simulink model "Link_B_org"  (Simulink 10.0)
settings: Solver=FixedStepAuto  StartTime=0.0  StopTime=15  FixedStep=1  RelTol=1e-3
model workspace (MAT data in the model file):
  Var : num (value not decoded)
libraries: Blocks_Lib x9
settings Model: Creator=aw5670  LastModifiedBy=bhisma
settings DataIOCC: LimitDataPoints=on
settings OptimizationCC: BlockReduction=off  BooleanDataType=off
settings DebuggingCC: SaveWithParameterizedLinksMsg=none  SignalResolutionControl=TryResolveAllWithWarning
settings HardwareCC: TargetUnknown=on
settings GRTTargetCC: GeneratePreprocessorConditionals=Disable all  CombineOutputUpdateFcns=on  GRTInterface=off
settings ConfigComp: CovExternalEMLEnable=off  CovSFcnEnable=off

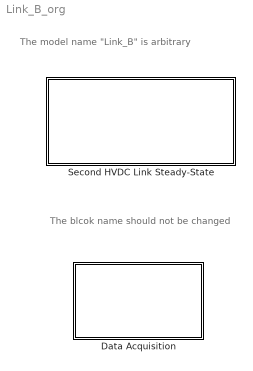
== system Link_B_org ==
  note: The model name "Link_B" is arbitrary
  note: The blcok name should not be changed
  Data Acquisition : Subsystem  mask{Ts=1}
      mask prompts: Ts "Sample time :"
      mask Display: disp('Open this block\nto visualize\nrecorded signals')
  Second HVDC Link Steady-State : Subsystem  mask(HVDC link steady-state model){NB_R=2, NOT_USED_3=, NOT_USED_4=, Pn_R=600, U1_R=[735, 0.0025, 0.01], U2_R=[200, 0.0025, 0.11], NOT_USED_0=DC current, NOT_USED_1=0, AMODE_ANGLE=5, LOCK_TAP_R=off, TCC_UDI0_MODE_R=off, ANGLE_R=[14.0, 17.0], Udi0_ref_R=280, TSTP_R=0.0125, TAP_R=[0.9375, 1.125], TAP_R_INI=1, Eac_R_INI=735, NB_I=2, NOT_USED_5=, NOT_USED_6=, Pn_I=600, U1_I=[735, 0.0025, 0.01], U2_I=[200, 0.0025, 0.11], C_MODE_I=DC voltage, GAMMA_REF=22, VSCHED=500, GMODE_ANGLE=17, NOT_USED_2=0, LOCK_TAP_I=off, TCC_UDI0_MODE_I=off, ANGLE_I=[20.0, 23.0], Udi0_ref_I=280, TSTP_I=0.0125, TAP_I=[0.9125, 1.0875], TAP_I_INI=1, Eac_I_INI=735, RDC=12.0 + 2*0.3, RCOMP=0.3, MC_MODE=Power, SLACK_ST=Rectifier, SETVAL_MW=100, SETVAL_kA=1, VCMODE=500*0.94, DELTI=0.2, Tap_pu_R_B=0.9875, Eac_R_B=741.9693, Udi0_R_B=276.1073, Tap_limited_R_B=0, alpha_R_B=16.7041, Idc_R_B=1, Vdc_R_B=512.3, Pdc_R_B=512.3, Pac_R_B=513.6333, Qac_R_B=201.3195, Tap_pu_I_B=1.0125, Eac_I_B=760.915, Udi0_I_B=276.166, Tap_limited_I_B=0, alpha_I_B=151.0016, gamma_I_B=21.5717, Vdc_I_B=499.7, Pdc_I_B=-499.7, Pac_I_B=-498.3667, Qac_I_B=237.2282, DC_iter_B=2, Ts=1}
      mask prompts: NB_R "Number of 6 pulse converter units in series"; NOT_USED_3 "AC bus name"; NOT_USED_4 "PQ load name"; Pn_R "Power (MVA)"; U1_R "Primary winding (AC side) parameters [V1 Ph-Ph(kVrms), R1(pu), L1(pu)]"; U2_R "Secondary winding (DC side) parameters [V2 Ph-Ph(kVrms), R2(pu), L2(pu)]"; NOT_USED_0 "Control mode"; NOT_USED_1 "not used"; AMODE_ANGLE "Minimum alpha (deg.)"; LOCK_TAP_R "Lock tap ratio"; TCC_UDI0_MODE_R "Udi0 control mode"; ANGLE_R "Angle range [min, max] (deg.)"; Udi0_ref_R "Udi0 reference (kV)"; TSTP_R "Tap step size (pu)"; TAP_R "Tap range [min, max] (pu)"; TAP_R_INI "Tap ratio (pu)"; Eac_R_INI "Primary AC voltage  (Ph-Ph(kVrms))"; NB_I "Number of 6 pulse converter units in series"; NOT_USED_5 "AC bus name"; NOT_USED_6 "PQ load name"; Pn_I "Power (MVA)"; U1_I "Primary winding (AC side) parameters [V1 Ph-Ph(kVrms), R1(pu), L1(pu)]"; U2_I "Secondary winding (DC side) parameters [V2 Ph-Ph(kVrms), R2(pu), L2(pu)]"; C_MODE_I "Control mode"; GAMMA_REF "Gamma reference (deg.)"; VSCHED "Voltage reference (kV)"; GMODE_ANGLE "Minimum gamma (deg.)"; NOT_USED_2 "Not used"; LOCK_TAP_I "Lock tap ratio"; TCC_UDI0_MODE_I "Udi0 control mode"; ANGLE_I "Angle range  [min, max] (deg.)"; Udi0_ref_I "Udi0 reference (kV)"; TSTP_I "Tap step size (pu)"; TAP_I "Tap range [min, max] (pu)"; TAP_I_INI "Tap ratio (pu)"; Eac_I_INI "Primary AC voltage  (Ph-Ph(kVrms))"; RDC "Total link resistance (ohm)"; RCOMP "Resistance between voltage measurement and converter (ohm)"; MC_MODE "Control mode"; SLACK_ST "Slack station"; SETVAL_MW "Power reference (MW)"; SETVAL_kA "Current reference (kA)"; VCMODE "Inverter DC voltage threshold in power control (kV)"; DELTI "Inverter current margin (kA)"; Tap_pu_R_B "Tap ratio (pu)"; Eac_R_B "Eac (kV)"; Udi0_R_B "Udi0 (kV)"; Tap_limited_R_B "Tap is limited"; alpha_R_B "Alpha (deg.)"; Idc_R_B "Idc (kA)"; Vdc_R_B "Vdc (kV)"; Pdc_R_B "Pdc (MW)"; Pac_R_B "Pac (MW)"; Qac_R_B "Qac (Mvar)"; Tap_pu_I_B "Tap ratio (pu)"; Eac_I_B "Eac (kV)"; Udi0_I_B "Udi0 (kV)"; Tap_limited_I_B "Tap is limited"; alpha_I_B "Alpha (deg.)"; gamma_I_B "Gamma (deg.)"; Vdc_I_B "Vdc (kV)"; Pdc_I_B "Pdc (MW)"; Pac_I_B "Pac (MW)"; Qac_I_B "Qac (Mvar)"; DC_iter_B "Iterations"; Ts "Sample time :"
      mask help: Implements a steady state model of a two terminal HVDC link for the DC load flow solution.
      mask init:
      | % History values 
      | Eac_R_B     = Eac_R_INI;
      | Eac_I_B     = Eac_I_INI;
      | TAPINI_R_B  = TAP_R_INI;
      | TAPINI_I_B  = TAP_I_INI;
      | 
      | % --- RECTIFIER ---
      | 
      | % Primary
      | V1_R = U1_R(1);
      | R1_R = U1_R(2);
      | L1_R = U1_R(3);
      | 
      | % Secondary
      | V2_R = U2_R(1);
      | R2_R = U2_R(2);
      | L2_R = U2_R(3);
      | 
      | % Nominal turn ratio (Usec/Uprim):
      | TR_R = V2_R/V1_R;
      | 
      | % Transformer reactance seen from secondary, per bridge [XC](ohm):
      | XC_R = (L1_R+L2_R)*V2_R^2/Pn_R;
      | 
      | % Transformer resistance seen from secondary, per bridge [RC](ohm):
      | RC_R = (R1_R+R2_R)* V2_R^2/Pn_R; 
      | 
      | % Tap Changer Control
      | ALFMIN_R=ANGLE_R(1);
      | ALFMAX_R=ANGLE_R(2);
      | 
      | TAPMN_R=TAP_R(1);
      | TAPMX_R=TAP_R(2);
      | 
      | % --- INVERTER ---
      | % Primary
      | V1_I = U1_I(1);
      | R1_I = U1_I(2);
      | L1_I = U1_I(3);
      | 
      | % Secondary
      | V2_I = U2_I(1);
      | R2_I = U2_I(2);
      | L2_I = U2_I(3);
      | 
      | % Nominal turn ratio (Usec/Uprim):
      | TR_I = V2_I/V1_I;
      | 
      | % Transformer reactance seen from secondary, per bridge [XC](ohm):
      | XC_I = (L1_I+L2_I)*V2_I^2/Pn_I;
      | 
      | % Transformer resistance seen from secondary, per bridge [RC](ohm):
      | RC_I = (R1_I+R2_I)* V2_I^2/Pn_I; 
      | 
      | % Pole Control
      | GC = C_MODE_I - 1;  % GC (0/1) is used in the model
      | 
      | % Tap Changer Control
      | GAMMIN_I=ANGLE_I(1);
      | GAMMAX_I=ANGLE_I(2);
      | 
      | TAPMN_I=TAP_I(1);
      | TAPMX_I=TAP_I(2);
      | 
      | DCVMIN_I   = VSCHED * (1 - TSTP_I);     %(kV)
      | DCVMAX_I   = VSCHED * (1 + TSTP_I);
      | 
      | % --- Master Control ---
      | MDC = MC_MODE - 1;     % MDC (0,1, or 2) used in the model 
      | 
      | if (MDC == 1)   
      |     SETVAL = SETVAL_MW;
      | elseif (MDC == 2)
      |     SETVAL = SETVAL_kA;
      | else
      |     SETVAL = 0;
      | end
      mask Help: web('HVDC_Link_SS_help.htm');
      mask TypeOptions NOT_USED_0: DC current
      mask Callback LOCK_TAP_R:
      | mode=get_param(gcb,'LOCK_TAP_R');
      | cb = get_param(gcb,'MaskEnables');
      | cb{11}='on'; cb{12}='on';
      | 
      | if strcmp(mode,'on')
      |  cb{11}='off';  % Udi0 control mode
      |  cb{12}='off';  % Angle range
      | end
      | 
      | set_param(gcb,'MaskEnables',cb);
      mask Callback TCC_UDI0_MODE_R:
      | mode=get_param(gcb,'TCC_UDI0_MODE_R');
      | cb = get_param(gcb,'MaskEnables');
      | cb{10}='on'; cb{12}='on'; cb{13}='off';
      | 
      | if strcmp(mode,'on')
      |  cb{12}='off';  % Angle range
      |  cb{10}='off';  % Lock the tap position
      |  cb{13}='on';  % Lock the tap position
      | end
      | 
      | set_param(gcb,'MaskEnables',cb);
      mask TypeOptions C_MODE_I: DC voltage | Gamma angle
      mask Callback C_MODE_I:
      | mode=get_param(gcb,'C_MODE_I');
      | cb = get_param(gcb,'MaskEnables');
      | cb{25}='on'; cb{26}='on'; cb{27}='on'; cb{31}='on';
      | 
      | if strcmp(mode,'Gamma angle')
      |  cb{26}='off';    % Voltage reference
      |  cb{27}='off';    % Minimum gamma
      |  cb{31}='off';    % Angle range (gamma_
      | else
      |  cb{25}='off';    % Gamma reference
      | end
      | 
      | set_param(gcb,'MaskEnables',cb);
      mask Callback LOCK_TAP_I:
      | mode=get_param(gcb,'LOCK_TAP_I');
      | cb = get_param(gcb,'MaskEnables');
      | cb{30}='on'; cb{31}='on';
      | 
      | if strcmp(mode,'on')
      |  cb{30}='off';  % Udi0 control mode
      |  cb{31}='off';  % Angle range
      | end
      | 
      | set_param(gcb,'MaskEnables',cb);
      mask Callback TCC_UDI0_MODE_I:
      | mode=get_param(gcb,'TCC_UDI0_MODE_I');
      | cb = get_param(gcb,'MaskEnables');
      | cb{29}='on'; cb{31}='on';  cb{32}='off';
      | 
      | if strcmp(mode,'on')
      |  cb{29}='off';  % Lock the tap position
      |  cb{31}='off';  % Angle range
      |  cb{32}='on';   % Udi0 reference
      | end
      | 
      | set_param(gcb,'MaskEnables',cb);
      mask TypeOptions MC_MODE: Blocked | Power | Current
      mask Callback MC_MODE:
      | mode=get_param(gcb,'MC_MODE');
      | cb = get_param(gcb,'MaskEnables');
      |  cb{40}='on'; cb{41}='on'; cb{42}='on'; cb{43}='on';
      | 
      | if strcmp(mode,'Current')
      |  cb{40}='off';     % Slack station
      |  cb{41}='off';     % Power reference
      |  cb{43}='off';     % Inverter DC ...
      | end
      | 
      | if strcmp(mode,'Power')
      |  cb{42}='off';     % Current reference
      | end
      | 
      | set_param(gcb,'MaskEnables',cb);
      | clear cb mode;
      mask TypeOptions SLACK_ST: Rectifier | Inverter
      mask DialogControl Update_tap_R Prompt: Update
      mask DialogControl Update_tap_R Callback:
      | set_param(gcb,'TAP_R_INI',[num2str(Tap_pu_R(end)), '  %Updated']);
      | 
      | % Reset output values
      | set_param(gcb,'Idc_R',[num2str(0)]);
      | set_param(gcb,'alpha_R',[num2str(0)]);
      | set_param(gcb,'Udi0_R',[num2str(0)]);
      | set_param(gcb,'Vdc_R',[num2str(0)]);
      | set_param(gcb,'Pac_R',[num2str(0)]);
      | set_param(gcb,'Qac_R',[num2str(0)]);
      | set_param(gcb,'Pdc_R',[num2str(0)]);
      mask DialogControl Update_tap_I Prompt: Update
      mask DialogControl Update_tap_I Callback:
      | set_param(gcb,'TAP_I_INI',[num2str(Tap_pu_I(end)), '  %Updated']);
      | 
      | % Reset output values
      | set_param(gcb,'gamma_I',[num2str(0)]);
      | set_param(gcb,'alpha_I',[num2str(0)]);
      | set_param(gcb,'Udi0_I',[num2str(0)]);
      | set_param(gcb,'Vdc_I',[num2str(0)]);
      | set_param(gcb,'Pdc_I',[num2str(0)]);
      | set_param(gcb,'Pac_I',[num2str(0)]);
      | set_param(gcb,'Qac_I',[num2str(0)]);
      mask DialogControl Container31 Prompt: Rectifier
      mask DialogControl Container33 Prompt: Inverter
      mask DialogControl Control4 Prompt: Compute and Update
      mask DialogControl Control4 Callback:
      | sim(gcs);
      | set_param(gcb,'DC_iter_B',[num2str(DC_iter_B(end))]);
      | % Rectifier
      | set_param(gcb,'Eac_R_B',[num2str(Eac_R_B(end))]);
      | set_param(gcb,'Tap_pu_R_B',[num2str(Tap_pu_R_B(end))]);
      | set_param(gcb,'Tap_limited_R_B',[num2str(Tap_limited_R_B(end))]);
      | set_param(gcb,'Idc_R_B',[num2str(Idc_R_B(end))]);
      | set_param(gcb,'alpha_R_B',[num2str(alpha_R_B(end))]);
      | set_param(gcb,'Udi0_R_B',[num2str(Udi0_R_B(end))]);
      | set_param(gcb,'Vdc_R_B',[num2str(Vdc_R_B(end))]);
      | set_param(gcb,'Pdc_R_B',[num2str(Pdc_R_B(end))]);
      | set_param(gcb,'Pac_R_B',[num2str(Pac_R_B(end))]);
      | set_param(gcb,'Qac_R_B',[num2str(Qac_R_B(end))]);
      | 
      | % Inverter
      | set_param(gcb,'Eac_I_B',[num2str(Eac_I_B(end))]);
      | set_param(gcb,'Tap_pu_I_B',[num2str(Tap_pu_I_B(end))]);
      | set_param(gcb,'Tap_limited_I_B',[num2str(Tap_limited_I_B(end))]);
      | set_param(gcb,'gamma_I_B',[num2str(gamma_I_B(end))]);
      | set_param(gcb,'alpha_I_B',[num2str(alpha_I_B(end))]);
      | set_param(gcb,'Udi0_I_B',[num2str(Udi0_I_B(end))]);
      | set_param(gcb,'Vdc_I_B',[num2str(Vdc_I_B(end))]);
      | set_param(gcb,'Pdc_I_B',[num2str(Pdc_I_B(end))]);
      | set_param(gcb,'Pac_I_B',[num2str(Pac_I_B(end))]);
      | set_param(gcb,'Qac_I_B',[num2str(Qac_I_B(end))]);
      mask Display: disp('Steady-state model\nof HVDC link\n\n(for DC load flow solution)')

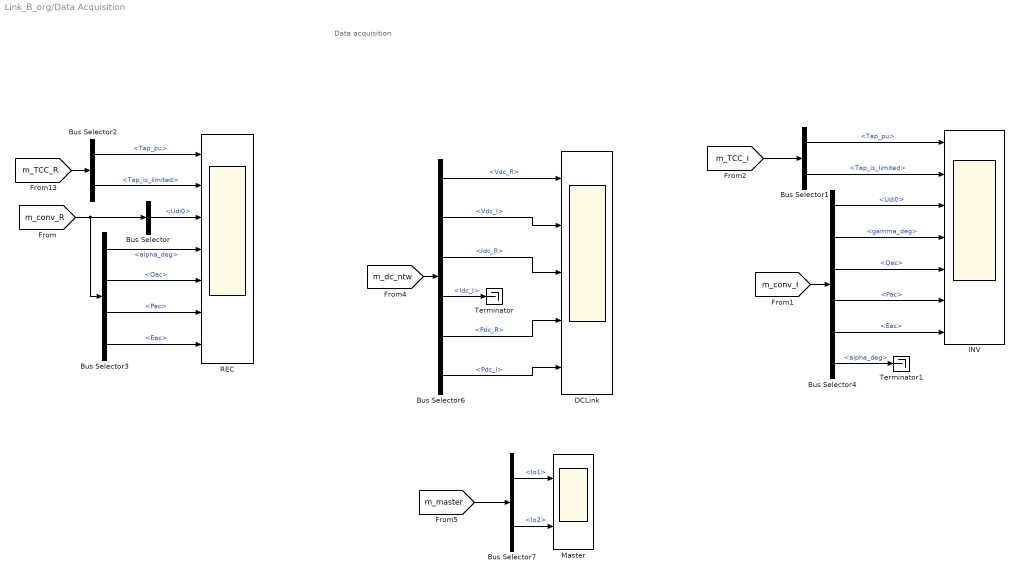
== system Link_B_org/Data Acquisition ==
  note: Data acquisition
  Bus Selector : BusSelector  OutputSignals=Udi0
  Bus Selector1 : BusSelector  OutputSignals=Tap_pu,Tap_is_limited
  Bus Selector2 : BusSelector  OutputSignals=Tap_pu,Tap_is_limited
  Bus Selector3 : BusSelector  OutputSignals=alpha_deg,Qac,Pac,Eac
  Bus Selector4 : BusSelector  OutputSignals=Udi0,gamma_deg,Qac,Pac,Eac,alpha_deg
  Bus Selector6 : BusSelector  OutputSignals=Vdc_R,Vdc_I,Idc_R,Idc_I,Pdc_R,Pdc_I
  Bus Selector7 : BusSelector  OutputSignals=Io1,Io2
  DCLink : Scope  NumInputPorts=5
  INV : Scope  NumInputPorts=7
  Master : Scope  NumInputPorts=2
  REC : Scope  NumInputPorts=7
  Terminator : Terminator
  Terminator1 : Terminator
  wires:
  Bus Selector1/1 -> INV/1  "<Tap_pu>"
  Bus Selector6/6 -> DCLink/5  "<Pdc_I>"
  Bus Selector6/5 -> DCLink/4  "<Pdc_R>"
  Bus Selector6/3 -> DCLink/3  "<Idc_R>"
  Bus Selector6/2 -> DCLink/2  "<Vdc_I>"
  Bus Selector1/2 -> INV/2  "<Tap_is_limited>"
  Bus Selector2/2 -> REC/2  "<Tap_is_limited>"
  Bus Selector7/2 -> Master/2  "<Io2>"
  Bus Selector7/1 -> Master/1  "<Io1>"
  [m_master] -> Bus Selector7/1
  Bus Selector/1 -> REC/3  "<Udi0>"
  [m_conv_R] -> Bus Selector/1, Bus Selector3/1
  Bus Selector3/2 -> REC/5  "<Qac>"
  Bus Selector3/1 -> REC/4  "<alpha_deg>"
  Bus Selector3/3 -> REC/6  "<Pac>"
  Bus Selector6/1 -> DCLink/1  "<Vdc_R>"
  Bus Selector2/1 -> REC/1  "<Tap_pu>"
  Bus Selector3/4 -> REC/7  "<Eac>"
  [m_conv_I] -> Bus Selector4/1
  [m_TCC_I] -> Bus Selector1/1
  [m_dc_ntw] -> Bus Selector6/1
  Bus Selector6/4 -> Terminator/1  "<Idc_I>"
  Bus Selector4/6 -> Terminator1/1  "<alpha_deg>"
  Bus Selector4/1 -> INV/3  "<Udi0>"
  Bus Selector4/2 -> INV/4  "<gamma_deg>"
  Bus Selector4/3 -> INV/5  "<Qac>"
  Bus Selector4/4 -> INV/6  "<Pac>"
  Bus Selector4/5 -> INV/7  "<Eac>"
  [m_TCC_R] -> Bus Selector2/1

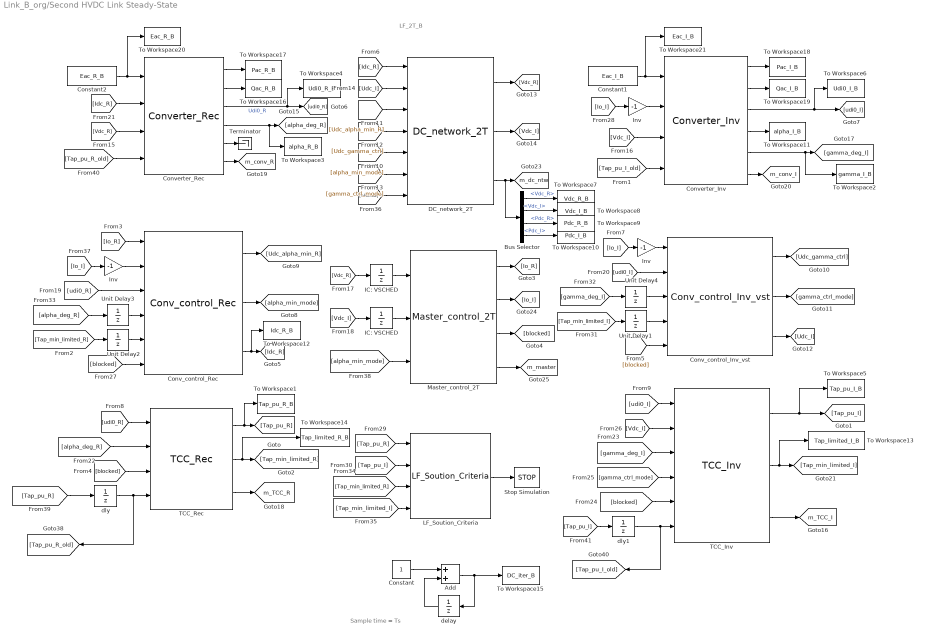
== system Link_B_org/Second HVDC Link Steady-State ==
  note: LF_2T_B
  note: Sample time = Ts
  " Inv " : Gain  Gain=-1
  Add : Sum
  Bus Selector : BusSelector  OutputSignals=Vdc_R,Vdc_I,Pdc_R,Pdc_I
  Constant : Constant
  Constant1 : Constant  Value=Eac_I_B
  Constant2 : Constant  Value=Eac_R_B
  Conv_control_Inv_vst : Blocks_Lib/Second HVDC Link Steady-State/Conv_control_Inv_vst  GC=GC  VSCHED=VSCHED  GMODE_ANGLE=GMODE_ANGLE  GAMMA_REF=GAMMA_REF  NB=NB_I  RC=RC_I  XC=XC_I
  Conv_control_Rec : Blocks_Lib/Second HVDC Link Steady-State/Conv_control_Rec  AMODE_ANGLE=AMODE_ANGLE  NB=NB_R  RC=RC_R  XC=XC_R
  Converter_Inv : Blocks_Lib/Second HVDC Link Steady-State/Converter_Inv  Pn=Pn_I  W1="[V1_I,  R1_I,  L1_I]"  W2=[V2_I, R2_I, L2_I]  TR=V2_I/V1_I  RC=(R1_I+R2_I)* V2_I^2/Pn_I;  XC=(L1_I+L2_I)*V2_I^2/Pn_I;  NB=NB_I
  Converter_Rec : Blocks_Lib/Second HVDC Link Steady-State/Converter_Rec  Pn=Pn_R  W1="[V1_R,  R1_R,  L1_R]"  W2="[V2_R,  R2_R,  L2_R]"  TR=V2_R/V1_R  RC=(R1_R+R2_R)* V2_R^2/Pn_R;  XC=(L1_R+L2_R)*V2_R^2/Pn_R;  NB=NB_R
  DC_network_2T : Blocks_Lib/Second HVDC Link Steady-State/DC_network_2T  RDC=RDC  RCOMP=RCOMP
  IC: VSCHED : UnitDelay  InitialCondition=VSCHED  SampleTime=-1  HasFrameUpgradeWarning=on
  "IC: VSCHED " : UnitDelay  InitialCondition=VSCHED  SampleTime=-1  HasFrameUpgradeWarning=on
  "Inv " : Gain  Gain=-1
  "Inv  " : Gain  Gain=-1
  LF_Soution_Criteria : Blocks_Lib/Second HVDC Link Steady-State/LF_Soution_Criteria
  Master_control_2T : Blocks_Lib/Second HVDC Link Steady-State/Master_control_2T  MDC=MDC  SLACK_ST=SLACK_ST  SETVAL=SETVAL  VCMODE=VCMODE
  Stop Simulation : Stop
  TCC_Inv : Blocks_Lib/Second HVDC Link Steady-State/TCC_Inv  LOCK_TAP=LOCK_TAP_I  TCC_UDI0_MODE=TCC_UDI0_MODE_I  Udi0_ref=Udi0_ref_I  TAPINI=TAPINI_I_B  TAPMN=TAPMN_I  TAPMX=TAPMX_I  TSTP=TSTP_I  GAMMIN=GAMMIN_I  GAMMAX=GAMMAX_I  DCVMIN=DCVMIN_I  DCVMAX=DCVMAX_I
      settings: AttributesFormatString=|
      | Udi0_min = (1-TSTP*0.75)* Udi0_ref
      | Udi0_max = (1+TSTP*0.75)* Udi0_ref
  TCC_Rec : Blocks_Lib/Second HVDC Link Steady-State/TCC_Rec  LOCK_TAP=LOCK_TAP_R  TCC_UDI0_MODE=TCC_UDI0_MODE_R  Udi0_ref=Udi0_ref_R  TAPINI=TAPINI_R_B  TAPMN=TAPMN_R  TAPMX=TAPMX_R  TSTP=TSTP_R  ALFMIN=ALFMIN_R  ALFMAX=ALFMAX_R
      settings: AttributesFormatString=|
      | Udi0_min = (1-TSTP*0.75)* Udi0_ref
      | Udi0_max = (1+TSTP*0.75)* Udi0_ref
  Terminator : Terminator
  To Workspace1 : ToWorkspace  VariableName=Tap_pu_R_B  SampleTime=-1
  To Workspace10 : ToWorkspace  VariableName=Pdc_I_B  SampleTime=-1
  To Workspace11 : ToWorkspace  VariableName=alpha_I_B  SampleTime=-1
  To Workspace12 : ToWorkspace  VariableName=Idc_R_B  SampleTime=-1
  To Workspace13 : ToWorkspace  VariableName=Tap_limited_I_B  SampleTime=-1
  To Workspace14 : ToWorkspace  VariableName=Tap_limited_R_B  SampleTime=-1
  To Workspace15 : ToWorkspace  VariableName=DC_iter_B  SampleTime=-1
  To Workspace16 : ToWorkspace  VariableName=Qac_R_B  SampleTime=-1
  To Workspace17 : ToWorkspace  VariableName=Pac_R_B  SampleTime=-1
  To Workspace18 : ToWorkspace  VariableName=Pac_I_B  SampleTime=-1
  To Workspace19 : ToWorkspace  VariableName=Qac_I_B  SampleTime=-1
  To Workspace2 : ToWorkspace  VariableName=gamma_I_B  SampleTime=-1
  To Workspace20 : ToWorkspace  VariableName=Eac_R_B  SampleTime=-1
  To Workspace21 : ToWorkspace  VariableName=Eac_I_B  SampleTime=-1
  To Workspace3 : ToWorkspace  VariableName=alpha_R_B  SampleTime=-1
  To Workspace4 : ToWorkspace  VariableName=Udi0_R_B  SampleTime=-1
  To Workspace5 : ToWorkspace  VariableName=Tap_pu_I_B  SampleTime=-1
  To Workspace6 : ToWorkspace  VariableName=Udi0_I_B  SampleTime=-1
  To Workspace7 : ToWorkspace  VariableName=Vdc_R_B  SampleTime=-1
  To Workspace8 : ToWorkspace  VariableName=Vdc_I_B  SampleTime=-1
  To Workspace9 : ToWorkspace  VariableName=Pdc_R_B  SampleTime=-1
  Unit Delay{1..4} (4 alike) : UnitDelay  SampleTime=-1  HasFrameUpgradeWarning=on
  delay : UnitDelay  SampleTime=Ts  HasFrameUpgradeWarning=on
      settings: AttributesFormatString=IC=%<InitialCondition>
  dly : UnitDelay  InitialCondition=TAPINI_R_B  SampleTime=-1  HasFrameUpgradeWarning=on
      settings: AttributesFormatString=IC=%<InitialCondition>
  dly1 : UnitDelay  InitialCondition=TAPINI_I_B  SampleTime=-1  HasFrameUpgradeWarning=on
      settings: AttributesFormatString=IC=%<InitialCondition>
  tag scope: m_TCC_I=global, m_TCC_R=global, m_conv_I=global, m_conv_R=global, m_dc_ntw=global, m_master=global
  wires:
  Conv_control_Rec/3 -> To Workspace12/1, [Idc_R]
  " Inv "/1 -> Conv_control_Rec/2
  DC_network_2T/3 -> Bus Selector/1, [m_dc_ntw]
  [Io_I] -> "Inv  "/1
  "Inv  "/1 -> Converter_Inv/2
  [Io_I] -> "Inv "/1
  "Inv "/1 -> Conv_control_Inv_vst/1
  Master_control_2T/4 -> [m_master]
  Master_control_2T/3 -> [blocked]
  Master_control_2T/2 -> [Io_I]
  Master_control_2T/1 -> [Io_R]
  [alpha_min_mode] -> Master_control_2T/3
  IC: VSCHED/1 -> Master_control_2T/1
  "IC: VSCHED "/1 -> Master_control_2T/2
  TCC_Inv/1 -> To Workspace5/1, [Tap_pu_I]
  TCC_Inv/2 -> [Tap_min_limited_I], To Workspace13/1
  TCC_Rec/2 -> [Tap_min_limited_R], To Workspace14/1
  [Io_R] -> Conv_control_Rec/1
  [blocked] -> TCC_Rec/3
  [Idc_R] -> DC_network_2T/1
  Converter_Rec/3 -> To Workspace4/1, [udi0_R]  "Udi0_R"
  Converter_Inv/3 -> To Workspace6/1, [udi0_I]
  [udi0_R] -> TCC_Rec/1
  [udi0_I] -> TCC_Inv/1
  [Tap_pu_R_old] -> Converter_Rec/4
  Conv_control_Rec/2 -> [alpha_min_mode]
  [alpha_min_mode] -> DC_network_2T/5
  Conv_control_Rec/1 -> [Udc_alpha_min_R]
  [Udc_alpha_min_R] -> DC_network_2T/3
  Conv_control_Inv_vst/1 -> [Udc_gamma_ctrl]
  [Udc_gamma_ctrl] -> DC_network_2T/4
  Conv_control_Inv_vst/2 -> [gamma_ctrl_mode]
  [gamma_ctrl_mode] -> DC_network_2T/6
  Conv_control_Inv_vst/3 -> [Udc_I]
  [Udc_I] -> DC_network_2T/2
  DC_network_2T/1 -> [Vdc_R]
  DC_network_2T/2 -> [Vdc_I]
  [Vdc_R] -> Converter_Rec/3
  [Vdc_R] -> IC: VSCHED/1
  [Vdc_I] -> "IC: VSCHED "/1
  [udi0_I] -> Conv_control_Inv_vst/2
  [Idc_R] -> Converter_Rec/2
  Converter_Rec/4 -> To Workspace3/1, [alpha_deg_R]
  Converter_Inv/4 -> To Workspace11/1
  Converter_Inv/5 -> [gamma_deg_I], To Workspace2/1
  [gamma_deg_I] -> TCC_Inv/3
  [blocked] -> TCC_Inv/5
  [gamma_ctrl_mode] -> TCC_Inv/4
  [Vdc_I] -> TCC_Inv/2
  Converter_Rec/5 -> Terminator/1
  [Vdc_I] -> Converter_Inv/3
  Converter_Rec/6 -> [m_conv_R]
  Converter_Inv/6 -> [m_conv_I]
  [Tap_pu_R] -> LF_Soution_Criteria/1
  Converter_Rec/1 -> To Workspace17/1
  Converter_Rec/2 -> To Workspace16/1
  Converter_Inv/1 -> To Workspace18/1
  Converter_Inv/2 -> To Workspace19/1
  [Tap_min_limited_I] -> Unit Delay1/1
  [blocked] -> Conv_control_Inv_vst/5
  Unit Delay1/1 -> Conv_control_Inv_vst/4
  TCC_Inv/3 -> [m_TCC_I]
  TCC_Rec/1 -> To Workspace1/1, [Tap_pu_R]
  TCC_Rec/3 -> [m_TCC_R]
  [Tap_pu_I] -> LF_Soution_Criteria/2
  [Tap_min_limited_R] -> LF_Soution_Criteria/3
  [Tap_min_limited_I] -> LF_Soution_Criteria/4
  LF_Soution_Criteria/1 -> Stop Simulation/1
  [blocked] -> DC_network_2T/7
  [blocked] -> Conv_control_Rec/6
  [udi0_R] -> Conv_control_Rec/3
  [Io_I] -> " Inv "/1
  [Tap_pu_I_old] -> Converter_Inv/4
  Bus Selector/1 -> To Workspace7/1  "<Vdc_R>"
  Bus Selector/4 -> To Workspace10/1  "<Pdc_I>"
  Bus Selector/3 -> To Workspace9/1  "<Pdc_R>"
  Bus Selector/2 -> To Workspace8/1  "<Vdc_I>"
  [Tap_min_limited_R] -> Unit Delay2/1
  Unit Delay2/1 -> Conv_control_Rec/5
  [alpha_deg_R] -> Unit Delay3/1
  Unit Delay3/1 -> Conv_control_Rec/4
  Unit Delay4/1 -> Conv_control_Inv_vst/3
  [gamma_deg_I] -> Unit Delay4/1
  dly/1 -> [Tap_pu_R_old], TCC_Rec/4
  [Tap_pu_R] -> dly/1
  dly1/1 -> [Tap_pu_I_old], TCC_Inv/6
  [Tap_pu_I] -> dly1/1
  [alpha_deg_R] -> TCC_Rec/2
  Constant2/1 -> To Workspace20/1, Converter_Rec/1
  Constant1/1 -> To Workspace21/1, Converter_Inv/1
  Add/1 -> To Workspace15/1, delay/1
  Constant/1 -> Add/1
  delay/1 -> Add/2
